simulink model "ret3"  (R2013a)
settings: Solver=ode45  StartTime=0.0  StopTime=4  RelTol=1e-3
values from neighbouring files (symbols this model uses):
  C = 1    [dcmsi.m]
  J = 1.1e-4    (= 0.00011)    [dcmsi.m]
  kt = 0.038    [dcmsi.m]
  La = 6.67e-4    (= 0.000667)    [dcmsi.m]
  Ra = 1.6    [dcmsi.m]
  V_source = 24*sqrt(2)    [dcmsi.m]
libraries: powerlib x14
settings Model: Creator=dello  LastModifiedBy=dello
settings DataIOCC: SignalLoggingSaveFormat=ModelDataLogs  SignalLoggingName=results
settings OptimizationCC: BlockReduction=off

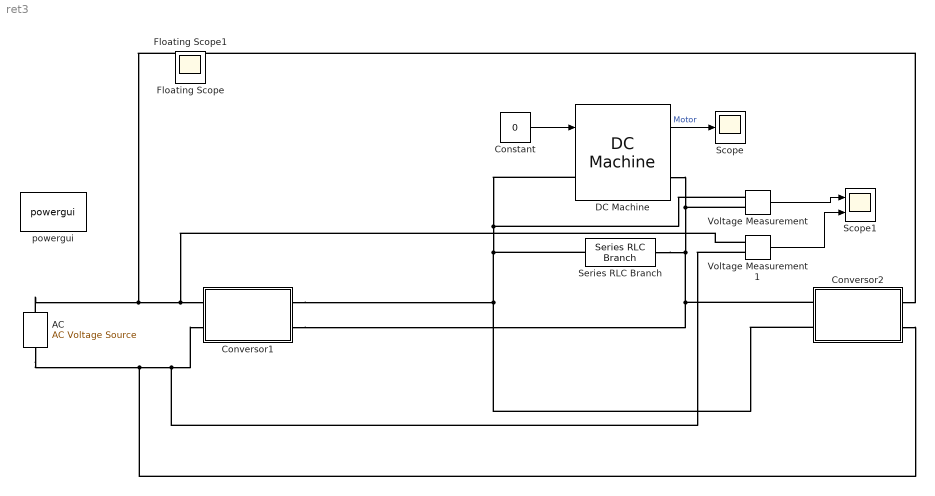
== system ret3 ==
  AC : powerlib/Electrical Sources/AC Voltage Source  Amplitude=V_source  Phase=0  Frequency=60  SampleTime=0  Measurements=Voltage
  Constant : Constant  Value=0
  Conversor1 : Subsystem
  Conversor2 : Subsystem
  DC Machine : powerlib/Machines/DC Machine  PresetModel=No  MechanicalLoad=Torque TL  FieldType=Permanent magnet  ShowDetailedParameters=on  RLa="[Ra  La]"  RLf="[ 240  120]"  Laf=1.8  MachineConstant=Torque constant (N.m/A)  Ke=1.8  Kt=kt  J=J  Bm=B  Tf=0  w0=0  Ifinit=1  TsPowergui=0  TsBlock=-1
  Scope : Scope
      settings: YMin=-700  YMax=700
  Scope1 : Scope  NumInputPorts=2
      settings: YMin=-35~-5  YMax=35~5
  Series RLC Branch : powerlib/Elements/Series RLC Branch  LConnTagsString=__new0  RConnTagsString=__new0  BranchType=C  Resistance=1  Inductance=1e-3  SetiL0=off  InitialCurrent=0  Capacitance=C  Setx0=off  InitialVoltage=0  Measurements=None
  Voltage Measurement : powerlib/Measurements/Voltage Measurement  PhasorSimulation=off  OutputType=Complex  PSBequivalent=0
  Voltage Measurement1 : powerlib/Measurements/Voltage Measurement  PhasorSimulation=off  OutputType=Complex  PSBequivalent=0
  powergui : powerlib/powergui  Priority=1  SimulationMode=Continuous  SolverType=Tustin  SampleTime=50e-6  frequency=60  SPID=off  DisableSnubberDevices=off  DisableRonSwitches=off  DisableVfSwitches=off  SwTol=0  Interpol=off  DisplayEquations=off  frequencyindice=0  Pbase=100e6  ErrMax=1e-4  Iterations=50  UnitsV=V  UnitsW=W  FunctionMessages=off  echomessages=off  HookPort=off  EnableUseOfTLC=off  x0status=blocks  RestoreLinks=warning  ResistiveCurrentMeasurement=off  Frange=[0:2:500]  Ylog=off  Xlog=on  ShowGrid=off  save=off  variable=ZData  ZoomFFT=off  StartTime=0.0  cycles=1  DisplayStyle=1  fundamental=60  FreqAxis=off  MaxFrequency=1000  frequencyindicesteady=1  RmsSteady=1  display=off  Ts=0  methode=off
  Floating Scope : Scope  NumInputPorts=8
      settings: Floating=on  TimeRange=0.03333333333333333  YMin=-5~-5~-5~-5~-5~-5~-5~-5  YMax=5~5~5~5~5~5~5~5  SaveName=diodes
  Floating Scope1 : Scope
      settings: Floating=on  TimeRange=0.03333333333333333  SaveName=simdata
  wires:
  Constant/1 -> DC Machine/1
  DC Machine/1 -> Scope/1  "Motor"
  Voltage Measurement/1 -> Scope1/1
  Voltage Measurement1/1 -> Scope1/2
  connections:
  Series RLC Branch/LConn1 -- DC Machine/LConn1 -- Voltage Measurement/LConn1 -- Conversor2/RConn2 -- Conversor1/RConn1
  DC Machine/RConn1 -- Conversor1/RConn2 -- Conversor2/RConn1 -- Series RLC Branch/RConn1 -- Voltage Measurement/LConn2
  AC/RConn1 -- Conversor2/LConn1 -- Voltage Measurement1/LConn1 -- Conversor1/LConn1
  AC/LConn1 -- Voltage Measurement1/LConn2 -- Conversor1/LConn2 -- Conversor2/LConn2

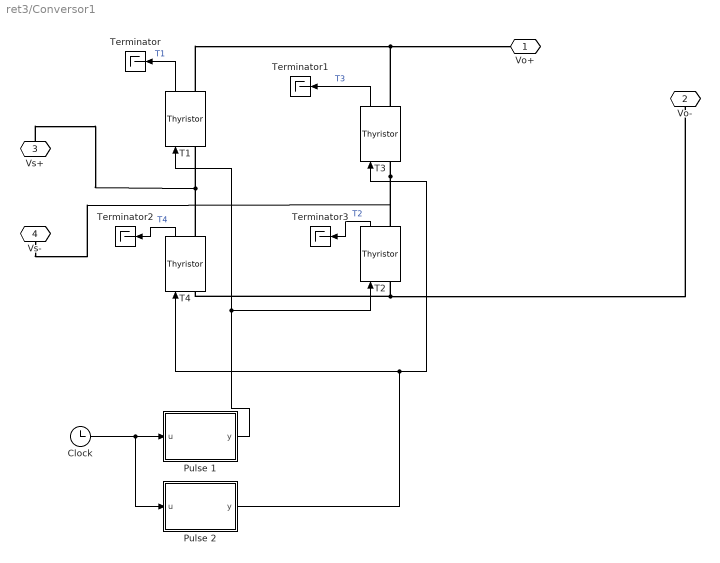
== system ret3/Conversor1 ==
  Clock : Clock
  Pulse 1 : MATLAB Function  TreatAsAtomicUnit=on
  Pulse 2 : MATLAB Function  TreatAsAtomicUnit=on
  T{1..4} (4 alike) : powerlib/Power Electronics/Thyristor  Ron=0.001  Lon=0  Vf=0.8  IC=0  Rs=500  Cs=250e-9  Measurements=on
  Terminator{,1..3} (4 alike) : Terminator
  Vo+ : PMIOPort  Port=1  Side=Right
  Vo- : PMIOPort  Port=2  Side=Right
  Vs+ : PMIOPort  Port=3  Side=Left
  Vs- : PMIOPort  Port=4  Side=Left
  wires:
  T4/1 -> Terminator2/1  "T4"
  T1/1 -> Terminator/1  "T1"
  T2/1 -> Terminator3/1  "T2"
  Pulse 2/1(y) -> T3/1, T4/1
  Pulse 1/1(y) -> T1/1, T2/1
  T3/1 -> Terminator1/1  "T3"
  Clock/1 -> Pulse 2/1(u), Pulse 1/1(u)
  connections:
  T4/RConn1 -- Vs+/RConn1 -- T1/LConn1
  T1/RConn1 -- Vo+/RConn1 -- T3/RConn1
  T3/LConn1 -- Vs-/RConn1 -- T2/RConn1
  T2/LConn1 -- Vo-/RConn1 -- T4/LConn1

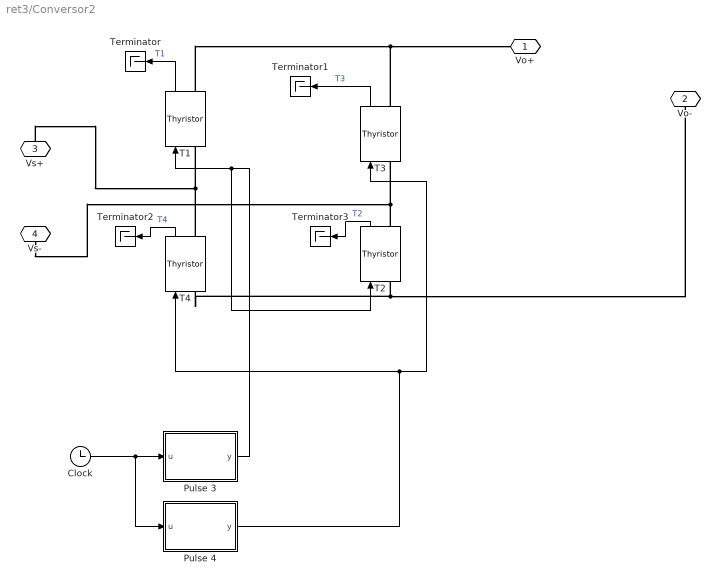
== system ret3/Conversor2 ==
  Clock : Clock
  Pulse 3 : MATLAB Function  TreatAsAtomicUnit=on
  Pulse 4 : MATLAB Function  TreatAsAtomicUnit=on
  T{1..4} (4 alike) : powerlib/Power Electronics/Thyristor  Ron=0.001  Lon=0  Vf=0.8  IC=0  Rs=500  Cs=250e-9  Measurements=on
  Terminator{,1..3} (4 alike) : Terminator
  Vo+ : PMIOPort  Port=1  Side=Right
  Vo- : PMIOPort  Port=2  Side=Right
  Vs+ : PMIOPort  Port=3  Side=Left
  Vs- : PMIOPort  Port=4  Side=Left
  wires:
  T4/1 -> Terminator2/1  "T4"
  T1/1 -> Terminator/1  "T1"
  T2/1 -> Terminator3/1  "T2"
  Pulse 4/1(y) -> T3/1, T4/1
  Pulse 3/1(y) -> T2/1, T1/1
  T3/1 -> Terminator1/1  "T3"
  Clock/1 -> Pulse 4/1(u), Pulse 3/1(u)
  connections:
  T4/RConn1 -- T1/LConn1 -- Vs+/RConn1
  T3/RConn1 -- T1/RConn1 -- Vo+/RConn1
  T2/RConn1 -- T3/LConn1 -- Vs-/RConn1
  T4/LConn1 -- T2/LConn1 -- Vo-/RConn1

== matlab function ret3/Conversor1/Pulse 1 ==
  data: u input; y output
function y = fcn(u)
    if u < 1
        alfa = 180;
    elseif u < 2
        alfa = 0;
    elseif u < 3;
        alfa = 180;
    else
        alfa = 0;
    end
    ti = mod(u*60*360, 360); 
    if ti >= alfa && ti <= alfa + 100
        a = 1;
    else
        a = 0;
    end
y = a;

== matlab function ret3/Conversor1/Pulse 2 ==
  data: u input; y output
function y = fcn(u)
    if u < 1
        alfa = 0;
    elseif u < 2
        alfa = 180;
    elseif u < 3
        alfa = 0;
    else
        alfa = 180;
    end
    ti = mod(u*60*360, 360); 
    if ti >= alfa && ti <= alfa + 100
        a = 1;
    else
        a = 0;
    end
y = a;

== matlab function ret3/Conversor2/Pulse 3 ==
  data: u input; y output
function y = fcn(u)
    if u < 2
        alfa = 180;
    elseif u < 3
        alfa = 0;
    else
        alfa = 0;
    end
    ti = mod(u*60*360, 360); 
    if ti >= alfa && ti <= alfa + 100
        a = 1;
    else
        a = 0;
    end
y = a;

== matlab function ret3/Conversor2/Pulse 4 ==
  data: u input; y output
function y = fcn(u)
    if u < 2
        alfa = 0;
    elseif u < 3
        alfa = 180;
    else
        alfa = 180;
    end
    ti = mod(u*60*360, 360); 
    if ti >= alfa && ti <= alfa + 100
        a = 1;
    else
        a = 0;
    end
y = a;
